simulink library "xpclib"  (Simulink 6.0)
settings: Solver=ode45  SolverMode=SingleTasking  StartTime=0.0  StopTime=10.0  RelTol=1e-3
values from neighbouring files (symbols this model uses):
  base = get_param( gcb, 'base' )    [maddiamondmm.m]    (also in maddiamondmm32frame.m; maddsmm16at.m; mdadsmm16at.m; mdiortddm64x0.m = hex2dec(addr(3:end)))
  block = find_system(bdroot,                          'FollowLinks', 'on',                          'LookUnderMasks', 'all',                          'MaskType', type )    [mdionipci6527.m]
  count = count + 1    (= 5)    [mdecodestate.m]
  port = get_param( gcb, 'port' )    [mdionipci6527.m]    (also in mdiortddm64x0.m = get_param(blocks{i}, 'port'))
undefined symbols (not defined in the file or in its folder): CIO, devid, DIO24, genixlib, get, handlers, irq, mbaseserialmask, mbwaudpmc, mdacbpcidas, mdiamondemeraldmask, mgenix, mmodemcontrol, mquamask, mrs232, msc150checks, mtargetboxleds, mtargetboxwatchdog, mxpccan, PCI, sizeof, vendid
libraries: xpclib x384, simulink x6
(part 4 of 7)

== system xpclib/RS232/Diamond/Emerald-MM8  ==
  Diamond Emerald-MM8 Serial : Subsystem  InitFcn=mdiamondemeraldmask(4,8)  TreatAsAtomicUnit=on  PropExecContextAcrossSSBoundary=on  mask(RS232 Send Receive){group=Board Setup, port=1, irqnum=5, saddr1=0x200, baud1=115200, parity1=None, ndata1=8, nstop1=1, fifomode1=16 deep, rlevel1=1, automode1=on, xmtfifosize1=1024, xmtdatatype1=8 bit uint null terminated, rcvfifosize1=1024, rcvmaxread1=1024, rcvminread1=1, rcvusedelim1=on, rcvdelim1=13, rcvdatatype1=count+16 bit uint, rcvsampletime1=-1, baud2=115200, parity2=None, ndata2=8, nstop2=1, fifomode2=16 deep, rlevel2=1, automode2=on, xmtfifosize2=1024, xmtdatatype2=8 bit uint null terminated, rcvfifosize2=1024, rcvmaxread2=1024, rcvminread2=1, rcvusedelim2=on, rcvdelim2=13, rcvdatatype2=count+16 bit uint, rcvsampletime2=-1, baud3=115200, parity3=None, ndata3=8, nstop3=1, fifomode3=16 deep, rlevel3=1, automode3=on, xmtfifosize3=1024, xmtdatatype3=8 bit uint null terminated, rcvfifosize3=1024, rcvmaxread3=1024, rcvminread3=1, rcvusedelim3=on, rcvdelim3=13, rcvdatatype3=count+16 bit uint, rcvsampletime3=-1, baud4=115200, parity4=None, ndata4=8, nstop4=1, fifomode4=16 deep, rlevel4=1, automode4=on, xmtfifosize4=1024, xmtdatatype4=8 bit uint null terminated, rcvfifosize4=1024, rcvmaxread4=1024, rcvminread4=1, rcvusedelim4=on, rcvdelim4=13, rcvdatatype4=count+16 bit uint, rcvsampletime4=-1, baud5=115200, parity5=None, ndata5=8, nstop5=1, fifomode5=16 deep, rlevel5=1, automode5=on, xmtfifosize5=1024, xmtdatatype5=8 bit uint null terminated, rcvfifosize5=1024, rcvmaxread5=1024, rcvminread5=1, rcvusedelim5=on, rcvdelim5=13, rcvdatatype5=count+16 bit uint, rcvsampletime5=-1, baud6=115200, parity6=None, ndata6=8, nstop6=1, fifomode6=16 deep, rlevel6=1, automode6=on, xmtfifosize6=1024, xmtdatatype6=8 bit uint null terminated, rcvfifosize6=1024, rcvmaxread6=1024, rcvminread6=1, rcvusedelim6=on, rcvdelim6=13, rcvdatatype6=count+16 bit uint, rcvsampletime6=-1, baud7=115200, parity7=None, ndata7=8, nstop7=1, fifomode7=16 deep, rlevel7=1, automode7=on, xmtfifosize7=1024, xmtdatatype7=8 bit uint null terminated, rcvfifosize7=1024, rcvmaxread7=1024, rcvminread7=1, rcvusedelim7=on, rcvdelim7=13, rcvdatatype7=count+16 bit uint, rcvsampletime7=-1, baud8=115200, parity8=None, ndata8=8, nstop8=1, fifomode8=16 deep, rlevel8=1, automode8=on, xmtfifosize8=1024, xmtdatatype8=8 bit uint null terminated, rcvfifosize8=1024, rcvmaxread8=1024, rcvminread8=1, rcvusedelim8=on, rcvdelim8=13, rcvdatatype8=count+16 bit uint, rcvsampletime8=-1}
      mask prompts: group "Parameter group:"; port "Port to modify:"; irqnum "IRQ number:"; saddr1 "Base address:"; baud1 "Baud rate:"; parity1 "Parity:"; ndata1 "Data bits:"; nstop1 "Stop bits:"; fifomode1 "Hardware fifo size:"; rlevel1 "Receive fifo interrupt level:"; automode1 "Auto RTS/CTS:"; xmtfifosize1 "Transmit software fifo size:"; xmtdatatype1 "Transmit fifo data type:"; rcvfifosize1 "Receive software fifo size:"; rcvmaxread1 "Receive maximum read:"; rcvminread1 "Receive minimum read:"; rcvusedelim1 "Read to delimiter:"; rcvdelim1 "Delimiter:"; rcvdatatype1 "Receive data type:"; rcvsampletime1 "Receive SampleTime:"; baud2 "Baud rate:"; parity2 "Parity:"; ndata2 "Data bits:"; nstop2 "Stop bits:"; fifomode2 "Hardware fifo size:"; rlevel2 "Receive fifo interrupt level:"; automode2 "Auto RTS/CTS:"; xmtfifosize2 "Transmit software fifo size:"; xmtdatatype2 "Transmit fifo data type:"; rcvfifosize2 "Receive software fifo size:"; rcvmaxread2 "Receive maximum read:"; rcvminread2 "Receive minimum read:"; rcvusedelim2 "Read to delimiter:"; rcvdelim2 "Delimiter:"; rcvdatatype2 "Receive data type:"; rcvsampletime2 "Receive SampleTime:"; baud3 "Baud rate:"; parity3 "Parity:"; ndata3 "Data bits:"; nstop3 "Stop bits:"; fifomode3 "Hardware fifo size:"; rlevel3 "Receive fifo interrupt level:"; automode3 "Auto RTS/CTS:"; xmtfifosize3 "Transmit software fifo size:"; xmtdatatype3 "Transmit fifo data type:"; rcvfifosize3 "Receive software fifo size:"; rcvmaxread3 "Receive maximum read:"; rcvminread3 "Receive minimum read:"; rcvusedelim3 "Read to delimiter:"; rcvdelim3 "Delimiter:"; rcvdatatype3 "Receive data type:"; rcvsampletime3 "Receive SampleTime:"; baud4 "Baud rate:"; parity4 "Parity:"; ndata4 "Data bits:"; nstop4 "Stop bits:"; fifomode4 "Hardware fifo size:"; rlevel4 "Receive fifo interrupt level:"; automode4 "Auto RTS/CTS:"; xmtfifosize4 "Transmit software fifo size:"; xmtdatatype4 "Transmit fifo data type:"; rcvfifosize4 "Receive software fifo size:"; rcvmaxread4 "Receive maximum read:"; rcvminread4 "Receive minimum read:"; rcvusedelim4 "Read to delimiter:"; rcvdelim4 "Delimiter:"; rcvdatatype4 "Receive data type:"; rcvsampletime4 "Receive SampleTime:"; baud5 "Baud rate:"; parity5 "Parity:"; ndata5 "Data bits:"; nstop5 "Stop bits:"; fifomode5 "Hardware fifo size:"; rlevel5 "Receive fifo interrupt level:"; automode5 "Auto RTS/CTS:"; xmtfifosize5 "Transmit software fifo size:"; xmtdatatype5 "Transmit fifo data type:"; rcvfifosize5 "Receive software fifo size:"; rcvmaxread5 "Receive maximum read:"; rcvminread5 "Receive minimum read:"; rcvusedelim5 "Read to delimiter:"; rcvdelim5 "Delimiter:"; rcvdatatype5 "Receive data type:"; rcvsampletime5 "Receive SampleTime:"; baud6 "Baud rate:"; parity6 "Parity:"; ndata6 "Data bits:"; nstop6 "Stop bits:"; fifomode6 "Hardware fifo size:"; rlevel6 "Receive fifo interrupt level:"; automode6 "Auto RTS/CTS:"; xmtfifosize6 "Transmit software fifo size:"; xmtdatatype6 "Transmit fifo data type:"; rcvfifosize6 "Receive software fifo size:"; rcvmaxread6 "Receive maximum read:"; rcvminread6 "Receive minimum read:"; rcvusedelim6 "Read to delimiter:"; rcvdelim6 "Delimiter:"; rcvdatatype6 "Receive data type:"; rcvsampletime6 "Receive SampleTime:"; baud7 "Baud rate:"; parity7 "Parity:"; ndata7 "Data bits:"; nstop7 "Stop bits:"; fifomode7 "Hardware fifo size:"; rlevel7 "Receive fifo interrupt level:"; automode7 "Auto RTS/CTS:"; xmtfifosize7 "Transmit software fifo size:"; xmtdatatype7 "Transmit fifo data type:"; rcvfifosize7 "Receive software fifo size:"; rcvmaxread7 "Receive maximum read:"; rcvminread7 "Receive minimum read:"; rcvusedelim7 "Read to delimiter:"; rcvdelim7 "Delimiter:"; rcvdatatype7 "Receive data type:"; rcvsampletime7 "Receive SampleTime:"; baud8 "Baud rate:"; parity8 "Parity:"; ndata8 "Data bits:"; nstop8 "Stop bits:"; fifomode8 "Hardware fifo size:"; rlevel8 "Receive fifo interrupt level:"; automode8 "Auto RTS/CTS:"; xmtfifosize8 "Transmit software fifo size:"; xmtdatatype8 "Transmit fifo data type:"; rcvfifosize8 "Receive software fifo size:"; rcvmaxread8 "Receive maximum read:"; rcvminread8 "Receive minimum read:"; rcvusedelim8 "Read to delimiter:"; rcvdelim8 "Delimiter:"; rcvdatatype8 "Receive data type:"; rcvsampletime8 "Receive SampleTime:"
      mask help:
      | Diamond Emerald MM-8
      | RS232 Send Receive Subsystem
      mask init:
      | addr = mdiamondemeraldmask( 1, 8 );
      | % addr(1) is base address, not used
      | baddr1 = addr{2};
      | baddr2 = addr{3};
      | baddr3 = addr{4};
      | baddr4 = addr{5};
      | baddr5 = addr{6};
      | baddr6 = addr{7};
      | baddr7 = addr{8};
      | baddr8 = addr{9};
      | istat = addr{10};
      | mdiamondemeraldmask( 3, 8 );
      mask Help: helpview(fullfile(docroot, 'mapfiles', 'xpc.map'), 'Baseboard_Serial_Subsystem')
      mask StyleString: popup(Board Setup|Basic Setup|Transmit Setup|Receive Setup),popup(1|2|3|4|5|6|7|8),edit,popup(0x100|0x140|0x180|0x1c0|0x200|0x240|0x280|0x2c0|0c300|0x340|0x380|0x3c0),popup(115200|57600|38400|19200|9600|4800|2400|1200|600|300|110),popup(None|Even|Odd|Mark|Space),popup(5|6|7|8),popup(1|2),popup(64 deep|16 deep|1 deep),popup(1|quarter full|half full|almost full),checkbox,edit,popup(count+32 bit int|count+32 bit uint|count+16 bit int|count+16 bit uint|8 bit int null terminated|8 bit uint null terminated),edit,edit,edit,checkbox,edit,popup(count+32 bit int|count+32 bit uint|count+16 bit int|count+16 bit uint|8 bit int null terminated|8 bit uint null terminated),edit,popup(115200|57600|38400|19200|9600|4800|2400|1200|600|300|110),popup(None|Even|Odd|Mark|Space),popup(5|6|7|8),popup(1|2),popup(64 deep|16 deep|1 deep),popup(1|quarter full|half full|almost full),checkbox,edit,popup(count+32 bit int|count+32 bit uint|count+16 bit int|count+16 bit uint|8 bit int null terminated|8 bit uint null terminated),edit,edit,edit,checkbox,edit,popup(count+32 bit int|count+32 bit uint|count+16 bit int|count+16 bit uint|8 bit int null terminated|8 bit uint null terminated),edit,popup(115200|57600|38400|19200|9600|4800|2400|1200|600|300|110),popup(None|Even|Odd|Mark|Space),popup(5|6|7|8),popup(1|2),popup(64 deep|16 deep|1 deep),popup(1|quarter full|half full|almost full),checkbox,edit,popup(count+32 bit int|count+32 bit uint|count+16 bit int|count+16 bit uint|8 bit int null terminated|8 bit uint null terminated),edit,edit,edit,checkbox,edit,popup(count+32 bit int|count+32 bit uint|count+16 bit int|count+16 bit uint|8 bit int null terminated|8 bit uint null terminated),edit,popup(115200|57600|38400|19200|9600|4800|2400|1200|600|300|110),popup(None|Even|Odd|Mark|Space),popup(5|6|7|8),popup(1|2),popup(64 deep|16 deep|1 deep),popup(1|quarter full|half full|almost full),checkbox,edit,popup(count+32 bit int|count+32 bit uint|count+16 bit int|count+16 bit uint|8 bit int null terminated|8 bit uint null terminated),edit,edit,edit,checkbox,edit,popup(count+32 bit int|count+32 bit uint|count+16 bit int|count+16 bit uint|8 bit int null terminated|8 bit uint null terminated),edit,popup(115200|57600|38400|19200|9600|4800|2400|1200|600|300|110),popup(None|Even|Odd|Mark|Space),popup(5|6|7|8),popup(1|2),popup(64 deep|16 deep|1 deep),popup(1|quarter full|half full|almost full),checkbox,edit,popup(count+32 bit int|count+32 bit uint|count+16 bit int|count+16 bit uint|8 bit int null terminated|8 bit uint null terminated),edit,edit,edit,checkbox,edit,popup(count+32 bit int|count+32 bit uint|count+16 bit int|count+16 bit uint|8 bit int null terminated|8 bit uint null terminated),edit,popup(115200|57600|38400|19200|9600|4800|2400|1200|600|300|110),popup(None|Even|Odd|Mark|Space),popup(5|6|7|8),popup(1|2),popup(64 deep|16 deep|1 deep),popup(1|quarter full|half full|almost full),checkbox,edit,popup(count+32 bit int|count+32 bit uint|count+16 bit int|count+16 bit uint|8 bit int null terminated|8 bit uint null terminated),edit,edit,edit,checkbox,edit,popup(count+32 bit int|count+32 bit uint|count+16 bit int|count+16 bit uint|8 bit int null terminated|8 bit uint null terminated),edit,popup(115200|57600|38400|19200|9600|4800|2400|1200|600|300|110),popup(None|Even|Odd|Mark|Space),popup(5|6|7|8),popup(1|2),popup(64 deep|16 deep|1 deep),popup(1|quarter full|half full|almost full),checkbox,edit,popup(count+32 bit int|count+32 bit uint|count+16 bit int|count+16 bit uint|8 bit int null terminated|8 bit uint null terminated),edit,edit,edit,checkbox,edit,popup(count+32 bit int|count+32 bit uint|count+16 bit int|count+16 bit uint|8 bit int null terminated|8 bit uint null terminated),edit,popup(115200|57600|38400|19200|9600|4800|2400|1200|600|300|110),popup(None|Even|Odd|Mark|Space),popup(5|6|7|8),popup(1|2),popup(64 deep|16 deep|1 deep),popup(1|quarter full|half full|almost full),checkbox,edit,popup(count+32 bit int|count+32 bit uint|count+16 bit int|count+16 bit uint|8 bit int null terminated|8 bit uint null terminated),edit,edit,edit,checkbox,edit,popup(count+32 bit int|count+32 bit uint|count+16 bit int|count+16 bit uint|8 bit int null terminated|8 bit uint null terminated),edit
      mask CallbackString:
      | mdiamondemeraldmask( 2, 8 );
      | |mdiamondemeraldmask( 2, 8 );||||||||||||||||||||||||||||||||||||||||||||||||||||||||||||||||||||||||||||||||||||||||||||||||||||||||||||||||||||||||||||||||||
      mask Display:
      | disp('Diamond\n\nEmerald\n\nRS232\nSend Receive');
      | port_label('input',1,'XMT1');
      | port_label('input',2,'XMT2');
      | port_label('input',3,'XMT3');
      | port_label('input',4,'XMT4');
      | port_label('input',5,'XMT5');
      | port_label('input',6,'XMT6');
      | port_label('input',7,'XMT7');
      | port_label('input',8,'XMT8');
      | port_label('output',1,'RCV1');
      | port_label('output',2,'RCV2');
      | port_label('output',3,'RCV3');
      | port_label('output',4,'RCV4');
      | port_label('output',5,'RCV5');
      | port_label('output',6,'RCV6');
      | port_label('output',7,'RCV7');
      | port_label('output',8,'RCV8');
  "Diamond Emerald-MM8 " : Subsystem  PropExecContextAcrossSSBoundary=on
  "Modem Control " : S-Function  InitFcn=mmodemcontrol(5);  FunctionName=modemcontrolemeraldmm  Parameters=addr, boardtype, rts, dtr, count  mask(Modem Control){port=1, rts=on, dtr=on, firstaddr=0x200}
      mask prompts: firstaddr "Configuration port address:"
      mask help:
      | Diamond Emerald-MM-8
      | Modem Control
      mask init:
      | count = 0;
      | boardtype = 6;
      | [maskdisplay, count, addr] = mmodemcontrol( 2, rts, dtr, boardtype, port, firstaddr );
      | addr = hex2dec( addr(3:end) );
      | set_param( gcb, 'MaskDisplay', maskdisplay );
      mask Help: helpview(fullfile(docroot, 'mapfiles', 'xpc.map'), 'Emerald_MODEM_Control')
      mask StyleString: popup(1|2|3|4|5|6|7|8),checkbox,checkbox,popup(0x100|0x140|0x180|0x1c0|0x200|0x240|0x280|0x2c0|0x300|0x340|0x380|0x3c0)
      mask Display: disp('Diamond\nEmerald-MM-8\nModem Control');port_label('input',1,'RTS');port_label('input',2,'DTR');
  "Modem Status " : S-Function  FunctionName=modemstatusemeraldmm  Parameters=addr, boardtype, cts, dsr, ring, dcd, count, sampletime  mask(Modem Status){port=1, cts=on, dsr=on, ring=on, dcd=on, sampletime=-1, firstaddr=0x200}
      mask prompts: ring "RI:"; firstaddr "Configuration port address:"
      mask help:
      | Diamond Emerald-MM-8
      | Modem Status
      mask init:
      | count = 0;
      | boardtype = 6;
      | [maskdisplay, count, addr] = mmodemstatus( 2, cts, dsr, ring, dcd, boardtype, port, firstaddr );
      | addr = hex2dec( addr(3:end) );
      | set_param( gcb, 'MaskDisplay', maskdisplay );
      mask Help: helpview(fullfile(docroot, 'mapfiles', 'xpc.map'), 'Emerald_MODEM_Status')
      mask StyleString: popup(1|2|3|4|5|6|7|8),checkbox,checkbox,checkbox,checkbox,edit,popup(0x100|0x140|0x180|0x1c0|0x200|0x240|0x280|0x2c0|0x300|0x340|0x380|0x3c0)
      mask Display: disp('Diamond\nEmerald-MM-8\nModem Status');port_label('output',1,'CTS');port_label('output',2,'DSR');port_label('output',3,'RI');port_label('output',4,'DCD');

== system xpclib/RS232/Mainboard/Baseboard Serial ==
  In1 : Inport  LatchInput=off
  In2 : Inport  Port=2  LatchInput=off
  Async Rate Transition{,1..3} (4 alike) : xpclib/Asynchronous Event/Async Rate Transition  sample_time=-1
  Enable TX 1 : xpclib/RS232/Mainboard/Baseboard Serial Internal  blocks/Enable TX   addr=baddr1
  Enable TX 2 : xpclib/RS232/Mainboard/Baseboard Serial Internal  blocks/Enable TX   addr=baddr2
  FIFO read 1 : xpclib/RS232/FIFO read   maxsize=1024  minsize=1  usedelimiter=on  delimiter=13  outputtype=count+16 bit uint  enable=off  enableout=off  sampletime=-1
  FIFO read 2 : xpclib/RS232/FIFO read   maxsize=1024  minsize=1  usedelimiter=on  delimiter=13  outputtype=count+16 bit uint  enable=off  enableout=off  sampletime=-1
  FIFO write 1 : xpclib/RS232/FIFO write   size=1024  inputtype=8 bit uint null terminated  present=on  sampletime=-1  id=XMT channel 1, IRQ 4
  FIFO write 2 : xpclib/RS232/FIFO write   size=1024  inputtype=8 bit uint null terminated  present=on  sampletime=-1  id=XMT channel 2, IRQ 4
  IRQ Source : xpclib/Asynchronous Event/IRQ Source  irqNo=4  preempt=off  b_type=None/Other  slot=-1
  RS232 ISR : Subsystem  TreatAsAtomicUnit=on  PropExecContextAcrossSSBoundary=on  mask(RS232 ISR){addr1=baddr1, addr2=baddr2}
      mask prompts: addr1 "First channel address:"; addr2 "Second channel address:"
      mask help:
      | Baseboard Serial
      | Interrupt Service Routine
      mask init:
      | baddr1 = addr1;
      | baddr2 = addr2;
      mask Display:
      | disp('Baseboard\nSerial\nISR');
      | port_label('input', 1, 'XMT1');
      | port_label('input', 2, 'XMT3');
      | port_label('output', 1, 'RCV1');
      | port_label('output', 2, 'RCV3');
  Setup1 : xpclib/RS232/Mainboard/Baseboard Serial Internal  blocks/Setup  baud=115200  width=8  nstop=1  parity=None  fmode=16 deep  rlevel=half full  ctsmode=on  addr=baddr1
  Setup2 : xpclib/RS232/Mainboard/Baseboard Serial Internal  blocks/Setup  baud=115200  width=8  nstop=1  parity=None  fmode=16 deep  rlevel=half full  ctsmode=off  addr=baddr2
  Out1 : Outport
  Out2 : Outport  Port=2
  wires:
  Async Rate Transition3/1 -> RS232 ISR/2(Xmt 2)
  FIFO write 2/2 -> Enable TX 2/1
  FIFO read 2/1 -> Out2/1
  Async Rate Transition1/1 -> FIFO read 2/1
  FIFO read 1/1 -> Out1/1
  Async Rate Transition/1 -> FIFO read 1/1
  In2/1 -> FIFO write 2/1
  FIFO write 2/1 -> Async Rate Transition3/1
  In1/1 -> FIFO write 1/1
  FIFO write 1/1 -> Async Rate Transition2/1
  RS232 ISR/2(Recv 2) -> Async Rate Transition1/1
  RS232 ISR/1(Recv 1) -> Async Rate Transition/1
  Async Rate Transition2/1 -> RS232 ISR/1(Xmt 1)
  IRQ Source/1 -> RS232 ISR/Trigger
  FIFO write 1/2 -> Enable TX 1/1

== system xpclib/RS232/Mainboard/Baseboard Serial Internal  blocks ==
  "Enable TX " : S-Function  FunctionName=sertxenablebase  Parameters=addr  mask(Enable TX Int){addr=0}
      mask prompts: addr "Base address:"
      mask help:
      | Baseboard Serial
      | Enable TX Interrupt
      mask init:
      | addr = hex2dec( addr(3:end) );
      mask Help: helpview(fullfile(docroot, 'mapfiles', 'xpc.map'), 'Baseboard_Enable_Int')
      mask Display:
      | disp('Baseboard\nSerial\nEnable TX Int');
      | port_label('input', 1, 'E');
  Filter Int Reason : S-Function  FunctionName=filterserint  Parameters=port, value  mask(Interrupt Source Filter){port=1, value=Receive data}
      mask prompts: value "Filter value:"
      mask help:
      | Baseboard
      | Interrupt Source Filter
      mask Help: helpview(fullfile(docroot, 'mapfiles', 'xpc.map'), 'Baseboard_Filter_Ints')
      mask StyleString: popup(1|2),popup(Receive data|Transmitter empty|Modem status change)
      mask Display:
      | disp('Baseboard\nSerial\nFilter Int Reason');
      | port_label('input', 1, 'S' );
      | port_label('output', 1, 'E' );
  Read HW FIFO : S-Function  FunctionName=serreadbase  Parameters=addr, flush  mask(Read Data Port){flush=on, addr=0}
      mask prompts: flush "Flush HW FIFO on startup"; addr "Base address:"
      mask help:
      | Baseboard
      | Read Data Port
      mask init:
      | addr = hex2dec( addr(3:end) );
      mask Help: helpview(fullfile(docroot, 'mapfiles', 'xpc.map'), 'Baseboard_Read_HW')
      mask Display:
      | disp('Baseboard\nSerial\nRead HW FIFO');
      | port_label('input', 1, 'E');
      | port_label('output', 1, 'D');
  Read Int Status : S-Function  FunctionName=iquerybase  Parameters=addr1, addr2  mask(Interrupt Query){addr1=0, addr2=0}
      mask prompts: addr1 "Base address 1"; addr2 "Base address 2"
      mask help:
      | Baseboard Serial
      | Interrupt Query
      mask init:
      | addr1 = hex2dec( addr1(3:end) );
      | addr2 = hex2dec( addr2(3:end) );
      mask Help: helpview(fullfile(docroot, 'mapfiles', 'xpc.map'), 'Baseboard_Interrupt_Query')
      mask Display:
      | disp('Baseboard\nSerial\nRead Int Status');
      | port_label('output', 1, 'S' );
  Setup : S-Function  FunctionName=sersetupbase  Parameters=addr, baud, width, nstop, parity, fmode, ctsmode, rlevel  mask(setup){baud=115200, width=8, nstop=1, parity=None, fmode=16 deep, rlevel=half full, ctsmode=off, addr=0}
      mask prompts: baud "Baud rate:"; width "Number of data bits:"; nstop "Number of stop bits:"; fmode "Fifo mode:"; rlevel "Receive trigger level:"; ctsmode "Enable auto RTS/CTS"; addr "Base Address:"
      mask help:
      | Baseboard
      | Serial
      | Setup
      mask init:
      | addr = hex2dec( addr(3:end) );
      mask Help: helpview(fullfile(docroot, 'mapfiles', 'xpc.map'), 'Baseboard_Setup')
      mask StyleString: popup(115200|57600|38400|19200|9600|4800|2400|1200|600|300|110),popup(5|6|7|8),popup(1|2),popup(None|Even|Odd|Mark|Space),popup(64 deep|16 deep|1 deep),popup(1|quarter full|half full|almost full),checkbox,edit
      mask Display: disp('Baseboard\nSerial\nSetup');
  Write HW FIFO : S-Function  FunctionName=serwritebase  Parameters=addr  mask(Write Data Port){addr=0}
      mask prompts: addr "Base address:"
      mask help:
      | Baseboard
      | Write Data Port
      mask init:
      | addr = hex2dec( addr(3:end) );
      mask Help: helpview(fullfile(docroot, 'mapfiles', 'xpc.map'), 'Baseboard_Write_HW')
      mask Display:
      | disp('Baseboard\nSerial\nWrite HW FIFO');
      | port_label('input', 1, 'D');
      | port_label('input', 2, 'E');

== system xpclib/RS232/Quatech/ESC-100 ==
  ESC-100 : Subsystem  InitFcn=mquamask(3)  TreatAsAtomicUnit=on  PropExecContextAcrossSSBoundary=on  mask(ESC-100 RS232 Send Receive){group=Board Setup, port=1, irqnum=7, slot=-1, baud1=19200, parity1=None, ndata1=8, nstop1=1, fifomode1=64 deep, rlevel1=half full, automode1=on, xmtfifosize1=1024, xmtdatatype1=8 bit uint null terminated, rcvfifosize1=1024, rcvmaxread1=1024, rcvminread1=1, rcvusedelim1=on, rcvdelim1=13, rcvdatatype1=count+16 bit uint, rcvsampletime1=-1, baud2=19200, parity2=None, ndata2=8, nstop2=1, fifomode2=64 deep, rlevel2=half full, automode2=on, xmtfifosize2=1024, xmtdatatype2=8 bit uint null terminated, rcvfifosize2=1024, rcvmaxread2=1024, rcvminread2=1, rcvusedelim2=on, rcvdelim2=13, rcvdatatype2=count+16 bit uint, rcvsampletime2=-1, baud3=19200, parity3=None, ndata3=8, nstop3=1, fifomode3=64 deep, rlevel3=half full, automode3=on, xmtfifosize3=1024, xmtdatatype3=8 bit uint null terminated, rcvfifosize3=1024, rcvmaxread3=1024, rcvminread3=1, rcvusedelim3=on, rcvdelim3=13, rcvdatatype3=count+16 bit uint, rcvsampletime3=-1, buad4=19200, parity4=None, ndata4=8, nstop4=1, fifomode4=64 deep, rlevel4=half full, automode4=on, xmtfifosize4=1024, xmtdatatype4=8 bit uint null terminated, rcvfifosize4=1024, rcvmaxread4=1024, rcvminread4=1, rcvusedelim4=on, rcvdelim4=13, rcvdatatype4=count+16 bit uint, rcvsampletime4=-1, baud5=19200, parity5=None, ndata5=8, nstop5=1, fifomode5=64 deep, rlevel5=half full, automode5=on, xmtfifosize5=1024, xmtdatatype5=8 bit uint null terminated, rcvfifosize5=1024, rcvmaxread5=1024, rcvminread5=1, rcvusedelim5=on, rcvdelim5=13, rcvdatatype5=count+16 bit uint, rcvsampletime5=-1, baud6=19200, parity6=None, ndata6=8, nstop6=1, fifomode6=64 deep, rlevel6=half full, automode6=on, xmtfifosize6=1024, xmtdatatype6=8 bit uint null terminated, rcvfifosize6=1024, rcvmaxread6=1024, rcvminread6=1, rcvusedelim6=on, rcvdelim6=13, rcvdatatype6=count+16 bit uint, rcvsampletime6=-1, baud7=19200, parity7=None, ndata7=8, nstop7=1, fifomode7=64 deep, rlevel7=half full, automode7=on, xmtfifosize7=1024, xmtdatatype7=8 bit uint null terminated, rcvfifosize7=1024, rcvmaxread7=1024, rcvminread7=1, rcvusedelim7=on, rcvdelim7=13, rcvdatatype7=count+16 bit uint, rcvsampletime7=-1, baud8=19200, parity8=None, ndata8=8, nstop8=1, fifomode8=64 deep, rlevel8=half full, automode8=on, xmtfifosize8=1024, xmtdatatype8=8 bit uint null terminated, rcvfifosize8=1024, rcvmaxread8=1024, rcvminread8=1, rcvusedelim8=on, rcvdelim8=13, rcvdatatype8=count+16 bit uint, rcvsampletime8=-1}
      mask prompts: group "Parameter group:"; port "Port to modify:"; irqnum "IRQ number:"; baud1 "Baud rate:"; parity1 "Parity:"; ndata1 "Data bits:"; nstop1 "Stop bits:"; fifomode1 "Hardware fifo size:"; rlevel1 "Receive fifo interrupt level:"; automode1 "Auto RTS/CTS:"; xmtfifosize1 "Transmit software fifo size:"; xmtdatatype1 "Transmit fifo data type:"; rcvfifosize1 "Receive software fifo size:"; rcvmaxread1 "Receive maximum read:"; rcvminread1 "Receive minimum read:"; rcvusedelim1 "Read to delimiter:"; rcvdelim1 "Delimiter:"; rcvdatatype1 "Receive data type:"; rcvsampletime1 "Receive SampleTime:"; baud2 "Baud rate:"; parity2 "Parity:"; ndata2 "Data bits:"; nstop2 "Stop bits:"; fifomode2 "Hardware fifo size:"; rlevel2 "Receive fifo interrupt level:"; automode2 "Auto RTS/CTS:"; xmtfifosize2 "Transmit software fifo size:"; xmtdatatype2 "Transmit fifo data type:"; rcvfifosize2 "Receive software fifo size:"; rcvmaxread2 "Receive maximum read:"; rcvminread2 "Receive minimum read:"; rcvusedelim2 "Read to delimiter:"; rcvdelim2 "Delimiter:"; rcvdatatype2 "Receive data type:"; rcvsampletime2 "Receive SampleTime:"; baud3 "Baud rate:"; parity3 "Parity:"; ndata3 "Data bits:"; nstop3 "Stop bits:"; fifomode3 "Hardware fifo size:"; rlevel3 "Receive fifo interrupt level:"; automode3 "Auto RTS/CTS:"; xmtfifosize3 "Transmit software fifo size:"; xmtdatatype3 "Transmit fifo data type:"; rcvfifosize3 "Receive software fifo size:"; rcvmaxread3 "Receive maximum read:"; rcvminread3 "Receive minimum read:"; rcvusedelim3 "Read to delimiter:"; rcvdelim3 "Delimiter:"; rcvdatatype3 "Receive data type:"; rcvsampletime3 "Receive SampleTime:"; buad4 "Baud rate:"; parity4 "Parity:"; ndata4 "Data bits:"; nstop4 "Stop bits:"; fifomode4 "Hardware fifo size:"; rlevel4 "Receive fifo interrupt level:"; automode4 "Auto RTS/CTS:"; xmtfifosize4 "Transmit software fifo size:"; xmtdatatype4 "Transmit fifo data type:"; rcvfifosize4 "Receive software fifo size:"; rcvmaxread4 "Receive maximum read:"; rcvminread4 "Receive minimum read:"; rcvusedelim4 "Read to delimiter:"; rcvdelim4 "Delimiter:"; rcvdatatype4 "Receive data type:"; rcvsampletime4 "Receive SampleTime:"; baud5 "Baud rate:"; parity5 "Parity:"; ndata5 "Data bits:"; nstop5 "Stop bits:"; fifomode5 "Hardware fifo size:"; rlevel5 "Receive fifo interrupt level:"; automode5 "Auto RTS/CTS:"; xmtfifosize5 "Transmit software fifo size:"; xmtdatatype5 "Transmit fifo data type:"; rcvfifosize5 "Receive software fifo size:"; rcvmaxread5 "Receive maximum read:"; rcvminread5 "Receive minimum read:"; rcvusedelim5 "Read to delimiter:"; rcvdelim5 "Delimiter:"; rcvdatatype5 "Receive data type:"; rcvsampletime5 "Receive SampleTime:"; baud6 "Baud rate:"; parity6 "Parity:"; ndata6 "Data bits:"; nstop6 "Stop bits:"; fifomode6 "Hardware fifo size:"; rlevel6 "Receive fifo interrupt level:"; automode6 "Auto RTS/CTS:"; xmtfifosize6 "Transmit software fifo size:"; xmtdatatype6 "Transmit fifo data type:"; rcvfifosize6 "Receive software fifo size:"; rcvmaxread6 "Receive maximum read:"; rcvminread6 "Receive minimum read:"; rcvusedelim6 "Read to delimiter:"; rcvdelim6 "Delimiter:"; rcvdatatype6 "Receive data type:"; rcvsampletime6 "Receive SampleTime:"; baud7 "Baud rate:"; parity7 "Parity:"; ndata7 "Data bits:"; nstop7 "Stop bits:"; fifomode7 "Hardware fifo size:"; rlevel7 "Receive fifo interrupt level:"; automode7 "Auto RTS/CTS:"; xmtfifosize7 "Transmit software fifo size:"; xmtdatatype7 "Transmit fifo data type:"; rcvfifosize7 "Receive software fifo size:"; rcvmaxread7 "Receive maximum read:"; rcvminread7 "Receive minimum read:"; rcvusedelim7 "Read to delimiter:"; rcvdelim7 "Delimiter:"; rcvdatatype7 "Receive data type:"; rcvsampletime7 "Receive SampleTime:"; baud8 "Baud rate:"; parity8 "Parity:"; ndata8 "Data bits:"; nstop8 "Stop bits:"; fifomode8 "Hardware fifo size:"; rlevel8 "Receive fifo interrupt level:"; automode8 "Auto RTS/CTS:"; xmtfifosize8 "Transmit software fifo size:"; xmtdatatype8 "Transmit fifo data type:"; rcvfifosize8 "Receive software fifo size:"; rcvmaxread8 "Receive maximum read:"; rcvminread8 "Receive minimum read:"; rcvusedelim8 "Read to delimiter:"; rcvdelim8 "Delimiter:"; rcvdatatype8 "Receive data type:"; rcvsampletime8 "Receive SampleTime:"
      mask help:
      | ESC-100
      | Quatech
      | RS232 Send Receive Subsystem
      mask init:
      | brdslot = slot;
      | mquamask( 1, 8 );
      mask Help: helpview(fullfile(docroot, 'mapfiles', 'xpc.map'), 'Quatech_Subsystem')
      mask StyleString: popup(Board Setup|Basic Setup|Transmit Setup|Receive Setup),popup(1|2|3|4|5|6|7|8),edit,edit,popup(921600|460800|230400|115200|57600|38400|19200|9600|4800|2400|1200|600|300|110),popup(None|Even|Odd|Mark|Space),popup(5|6|7|8),popup(1|2),popup(64 deep|16 deep|1 deep),popup(1|quarter full|half full|almost full),checkbox,edit,popup(count+32 bit int|count+32 bit uint|count+16 bit int|count+16 bit uint|8 bit int null terminated|8 bit uint null terminated),edit,edit,edit,checkbox,edit,popup(count+32 bit int|count+32 bit uint|count+16 bit int|count+16 bit uint|8 bit int null terminated|8 bit uint null terminated),edit,popup(921600|460800|230400|115200|57600|38400|19200|9600|4800|2400|1200|600|300|110),popup(None|Even|Odd|Mark|Space),popup(5|6|7|8),popup(1|2),popup(64 deep|16 deep|1 deep),popup(1|quarter full|half full|almost full),checkbox,edit,popup(count+32 bit int|count+32 bit uint|count+16 bit int|count+16 bit uint|8 bit int null terminated|8 bit uint null terminated),edit,edit,edit,checkbox,edit,popup(count+32 bit int|count+32 bit uint|count+16 bit int|count+16 bit uint|8 bit int null terminated|8 bit uint null terminated),edit,popup(921600|460800|230400|115200|57600|38400|19200|9600|4800|2400|1200|600|300|110),popup(None|Even|Odd|Mark|Space),popup(5|6|7|8),popup(1|2),popup(64 deep|16 deep|1 deep),popup(1|quarter full|half full|almost full),checkbox,edit,popup(count+32 bit int|count+32 bit uint|count+16 bit int|count+16 bit uint|8 bit int null terminated|8 bit uint null terminated),edit,edit,edit,checkbox,edit,popup(count+32 bit int|count+32 bit uint|count+16 bit int|count+16 bit uint|8 bit int null terminated|8 bit uint null terminated),edit,popup(921600|460800|230400|115200|57600|38400|19200|9600|4800|2400|1200|600|300|110),popup(None|Even|Odd|Mark|Space),popup(5|6|7|8),popup(1|2),popup(64 deep|16 deep|1 deep),popup(1|quarter full|half full|almost full),checkbox,edit,popup(count+32 bit int|count+32 bit uint|count+16 bit int|count+16 bit uint|8 bit int null terminated|8 bit uint null terminated),edit,edit,edit,checkbox,edit,popup(count+32 bit int|count+32 bit uint|count+16 bit int|count+16 bit uint|8 bit int null terminated|8 bit uint null terminated),edit,popup(921600|460800|230400|115200|57600|38400|19200|9600|4800|2400|1200|600|300|110),popup(None|Even|Odd|Mark|Space),popup(5|6|7|8),popup(1|2),popup(64 deep|16 deep|1 deep),popup(1|quarter full|half full|almost full),checkbox,edit,popup(count+32 bit int|count+32 bit uint|count+16 bit int|count+16 bit uint|8 bit int null terminated|8 bit uint null terminated),edit,edit,edit,checkbox,edit,popup(count+32 bit int|count+32 bit uint|count+16 bit int|count+16 bit uint|8 bit int null terminated|8 bit uint null terminated),edit,popup(921600|460800|230400|115200|57600|38400|19200|9600|4800|2400|1200|600|300|110),popup(None|Even|Odd|Mark|Space),popup(5|6|7|8),popup(1|2),popup(64 deep|16 deep|1 deep),popup(1|quarter full|half full|almost full),checkbox,edit,popup(count+32 bit int|count+32 bit uint|count+16 bit int|count+16 bit uint|8 bit int null terminated|8 bit uint null terminated),edit,edit,edit,checkbox,edit,popup(count+32 bit int|count+32 bit uint|count+16 bit int|count+16 bit uint|8 bit int null terminated|8 bit uint null terminated),edit,popup(921600|460800|230400|115200|57600|38400|19200|9600|4800|2400|1200|600|300|110),popup(None|Even|Odd|Mark|Space),popup(5|6|7|8),popup(1|2),popup(64 deep|16 deep|1 deep),popup(1|quarter full|half full|almost full),checkbox,edit,popup(count+32 bit int|count+32 bit uint|count+16 bit int|count+16 bit uint|8 bit int null terminated|8 bit uint null terminated),edit,edit,edit,checkbox,edit,popup(count+32 bit int|count+32 bit uint|count+16 bit int|count+16 bit uint|8 bit int null terminated|8 bit uint null terminated),edit,popup(921600|460800|230400|115200|57600|38400|19200|9600|4800|2400|1200|600|300|110),popup(None|Even|Odd|Mark|Space),popup(5|6|7|8),popup(1|2),popup(64 deep|16 deep|1 deep),popup(1|quarter full|half full|almost full),checkbox,edit,popup(count+32 bit int|count+32 bit uint|count+16 bit int|count+16 bit uint|8 bit int null terminated|8 bit uint null terminated),edit,edit,edit,checkbox,edit,popup(count+32 bit int|count+32 bit uint|count+16 bit int|count+16 bit uint|8 bit int null terminated|8 bit uint null terminated),edit
      mask CallbackString:
      | mquamask( 2, 8 );
      | |mquamask( 2, 8 );||||||||||||||||||||||||||||||||||||||||||||||||||||||||||||||||||||||||||||||||||||||||||||||||||||||||||||||||||||||||||||||||||
      mask Display:
      | disp('ESC-100\n\nRS232\n\nSend Receive');
      | port_label( 'input', 1, 'XMT1' );
      | port_label( 'input', 2, 'XMT2' );
      | port_label( 'input', 3, 'XMT3' );
      | port_label( 'input', 4, 'XMT4' );
      | port_label( 'input', 5, 'XMT5' );
      | port_label( 'input', 6, 'XMT6' );
      | port_label( 'input', 7, 'XMT7' );
      | port_label( 'input', 8, 'XMT8' );
      | port_label( 'output', 1, 'RCV1' );
      | port_label( 'output', 2, 'RCV2' );
      | port_label( 'output', 3, 'RCV3' );
      | port_label( 'output', 4, 'RCV4' );
      | port_label( 'output', 5, 'RCV5' );
      | port_label( 'output', 6, 'RCV6' );
      | port_label( 'output', 7, 'RCV7' );
      | port_label( 'output', 8, 'RCV8' );
  ESC-100 Internal blocks : Subsystem  PropExecContextAcrossSSBoundary=on
  Modem Control : S-Function  InitFcn=mmodemcontrol(3)  FunctionName=modemcontrolqua  Parameters=slot, port, boardtype, rts, dtr, count  mask(ESC-100 Modem Control){port=1, rts=on, dtr=on, slot=-1}
      mask prompts: slot "PCI slot: (-1 for autosearch)"
      mask help:
      | ESC-100
      | Quatech
      | Modem Control
      mask init:
      | count = 0;
      | boardtype = 2;
      | [maskdisplay, count] = mmodemcontrol( 2, rts, dtr, boardtype, 0, 0 );
      | set_param( gcb, 'MaskDisplay', maskdisplay );
      mask Help: helpview(fullfile(docroot, 'mapfiles', 'xpc.map'), 'Quatech_MODEM_Control')
      mask StyleString: popup(1|2|3|4|5|6|7|8),checkbox,checkbox,edit
      mask Display: disp('ESC-100\nQuatech\nModem Control');port_label('input',1,'RTS');port_label('input',2,'DTR');
  Modem Status : S-Function  FunctionName=modemstatusqua  Parameters=slot, port, boardtype, cts, dsr, ring, dcd, count, sampletime  mask(Modem Status){port=1, cts=on, dsr=on, ring=on, dcd=on, sampletime=-1, slot=-1}
      mask prompts: ring "RI:"; slot "PCI slot: (-1 for autosearch)"
      mask help:
      | ESC-100
      | Quatech
      | Modem Status
      mask init:
      | count = 0;
      | boardtype = 2;
      | [maskdisplay, count] = mmodemstatus( 2, cts, dsr, ring, dcd, boardtype );
      | set_param( gcb, 'MaskDisplay', maskdisplay );
      mask Help: helpview(fullfile(docroot, 'mapfiles', 'xpc.map'), 'Quatech_MODEM_Status')
      mask StyleString: popup(1|2|3|4|5|6|7|8),checkbox,checkbox,checkbox,checkbox,edit,edit
      mask Display: disp('ESC-100\nQuatech\nModem Status');port_label('output',1,'CTS');port_label('output',2,'DSR');port_label('output',3,'RI');port_label('output',4,'DCD');

== system xpclib/RS232/Quatech/QSC-100 ==
  Modem Control : S-Function  InitFcn=mmodemcontrol(3)  FunctionName=modemcontrolqua  Parameters=slot, port, boardtype, rts, dtr, count  mask(QSC-100 Modem Control){port=1, rts=on, dtr=on, slot=-1}
      mask prompts: slot "PCI slot: (-1 for autosearch)"
      mask help:
      | QSC-100
      | Quatech
      | Modem Control
      mask init:
      | count = 0;
      | boardtype = 1;
      | [maskdisplay, count] = mmodemcontrol( 2, rts, dtr, boardtype, 0, 0 );
      | set_param( gcb, 'MaskDisplay', maskdisplay );
      mask Help: helpview(fullfile(docroot, 'mapfiles', 'xpc.map'), 'Quatech_MODEM_Control')
      mask StyleString: popup(1|2|3|4),checkbox,checkbox,edit
      mask Display: disp('QSC-100\nQuatech\nModem Control');port_label('input',1,'RTS');port_label('input',2,'DTR');
  Modem Status : S-Function  FunctionName=modemstatusqua  Parameters=slot, port, boardtype, cts, dsr, ring, dcd, count, sampletime  mask(Modem Status){port=1, cts=on, dsr=on, ring=on, dcd=on, sampletime=-1, slot=-1}
      mask prompts: ring "RI:"; slot "PCI slot: (-1 for autosearch)"
      mask help:
      | QSC-100
      | Quatech
      | Modem Status
      mask init:
      | count = 0;
      | boardtype = 1;
      | [maskdisplay, count] = mmodemstatus( 2, cts, dsr, ring, dcd, boardtype );
      | set_param( gcb, 'MaskDisplay', maskdisplay );
      mask Help: helpview(fullfile(docroot, 'mapfiles', 'xpc.map'), 'Quatech_MODEM_Status')
      mask StyleString: popup(1|2|3|4),checkbox,checkbox,checkbox,checkbox,edit,edit
      mask Display: disp('QSC-100\nQuatech\nModem Status');port_label('output',1,'CTS');port_label('output',2,'DSR');port_label('output',3,'RI');port_label('output',4,'DCD');
  QSC-100 : Subsystem  InitFcn=mquamask(3)  TreatAsAtomicUnit=on  PropExecContextAcrossSSBoundary=on  mask(QSC-100 RS232 Send Receive){group=Transmit Setup, port=1, irqnum=7, slot=-1, baud1=115200, parity1=None, ndata1=8, nstop1=1, fifomode1=64 deep, rlevel1=half full, automode1=on, xmtfifosize1=1024, xmtdatatype1=8 bit uint null terminated, rcvfifosize1=1024, rcvmaxread1=1024, rcvminread1=1, rcvusedelim1=on, rcvdelim1=13, rcvdatatype1=count+16 bit uint, rcvsampletime1=-1, baud2=115200, parity2=None, ndata2=8, nstop2=1, fifomode2=64 deep, rlevel2=half full, automode2=on, xmtfifosize2=1024, xmtdatatype2=8 bit uint null terminated, rcvfifosize2=1024, rcvmaxread2=1024, rcvminread2=1, rcvusedelim2=on, rcvdelim2=13, rcvdatatype2=count+16 bit uint, rcvsampletime2=-1, baud3=115200, parity3=None, ndata3=8, nstop3=1, fifomode3=64 deep, rlevel3=half full, automode3=on, xmtfifosize3=1024, xmtdatatype3=8 bit uint null terminated, rcvfifosize3=1024, rcvmaxread3=1024, rcvminread3=1, rcvusedelim3=on, rcvdelim3=13, rcvdatatype3=count+16 bit uint, rcvsampletime3=-1, buad4=115200, parity4=None, ndata4=8, nstop4=1, fifomode4=64 deep, rlevel4=half full, automode4=on, xmtfifosize4=1024, xmtdatatype4=8 bit uint null terminated, rcvfifosize4=1024, rcvmaxread4=1024, rcvminread4=1, rcvusedelim4=on, rcvdelim4=13, rcvdatatype4=count+16 bit uint, rcvsampletime4=-1}
      mask prompts: group "Parameter group:"; port "Port to modify:"; irqnum "IRQ number:"; baud1 "Baud rate:"; parity1 "Parity:"; ndata1 "Data bits:"; nstop1 "Stop bits:"; fifomode1 "Hardware fifo size:"; rlevel1 "Receive fifo interrupt level:"; automode1 "Auto RTS/CTS:"; xmtfifosize1 "Transmit software fifo size:"; xmtdatatype1 "Transmit fifo data type:"; rcvfifosize1 "Receive software fifo size:"; rcvmaxread1 "Receive maximum read:"; rcvminread1 "Receive minimum read:"; rcvusedelim1 "Read to delimiter:"; rcvdelim1 "Delimiter:"; rcvdatatype1 "Receive data type:"; rcvsampletime1 "Receive SampleTime:"; baud2 "Baud rate:"; parity2 "Parity:"; ndata2 "Data bits:"; nstop2 "Stop bits:"; fifomode2 "Hardware fifo size:"; rlevel2 "Receive fifo interrupt level:"; automode2 "Auto RTS/CTS:"; xmtfifosize2 "Transmit software fifo size:"; xmtdatatype2 "Transmit fifo data type:"; rcvfifosize2 "Receive software fifo size:"; rcvmaxread2 "Receive maximum read:"; rcvminread2 "Receive minimum read:"; rcvusedelim2 "Read to delimiter:"; rcvdelim2 "Delimiter:"; rcvdatatype2 "Receive data type:"; rcvsampletime2 "Receive SampleTime:"; baud3 "Baud rate:"; parity3 "Parity:"; ndata3 "Data bits:"; nstop3 "Stop bits:"; fifomode3 "Hardware fifo size:"; rlevel3 "Receive fifo interrupt level:"; automode3 "Auto RTS/CTS:"; xmtfifosize3 "Transmit software fifo size:"; xmtdatatype3 "Transmit fifo data type:"; rcvfifosize3 "Receive software fifo size:"; rcvmaxread3 "Receive maximum read:"; rcvminread3 "Receive minimum read:"; rcvusedelim3 "Read to delimiter:"; rcvdelim3 "Delimiter:"; rcvdatatype3 "Receive data type:"; rcvsampletime3 "Receive SampleTime:"; buad4 "Baud rate:"; parity4 "Parity:"; ndata4 "Data bits:"; nstop4 "Stop bits:"; fifomode4 "Hardware fifo size:"; rlevel4 "Receive fifo interrupt level:"; automode4 "Auto RTS/CTS:"; xmtfifosize4 "Transmit software fifo size:"; xmtdatatype4 "Transmit fifo data type:"; rcvfifosize4 "Receive software fifo size:"; rcvmaxread4 "Receive maximum read:"; rcvminread4 "Receive minimum read:"; rcvusedelim4 "Read to delimiter:"; rcvdelim4 "Delimiter:"; rcvdatatype4 "Receive data type:"; rcvsampletime4 "Receive SampleTime:"
      mask help:
      | QSC-100
      | Quatech
      | RS232 Send Receive Subsystem
      mask init:
      | brdslot = slot;
      | mquamask( 1, 4 );
      mask Help: helpview(fullfile(docroot, 'mapfiles', 'xpc.map'), 'Quatech_Subsystem')
      mask StyleString: popup(Board Setup|Basic Setup|Transmit Setup|Receive Setup),popup(1|2|3|4),edit,edit,popup(921600|460800|230400|115200|57600|38400|19200|9600|4800|2400|1200|600|300|110),popup(None|Even|Odd|Mark|Space),popup(5|6|7|8),popup(1|2),popup(64 deep|16 deep|1 deep),popup(1|quarter full|half full|almost full),checkbox,edit,popup(count+32 bit int|count+32 bit uint|count+16 bit int|count+16 bit uint|8 bit int null terminated|8 bit uint null terminated),edit,edit,edit,checkbox,edit,popup(count+32 bit int|count+32 bit uint|count+16 bit int|count+16 bit uint|8 bit int null terminated|8 bit uint null terminated),edit,popup(921600|460800|230400|115200|57600|38400|19200|9600|4800|2400|1200|600|300|110),popup(None|Even|Odd|Mark|Space),popup(5|6|7|8),popup(1|2),popup(64 deep|16 deep|1 deep),popup(1|quarter full|half full|almost full),checkbox,edit,popup(count+32 bit int|count+32 bit uint|count+16 bit int|count+16 bit uint|8 bit int null terminated|8 bit uint null terminated),edit,edit,edit,checkbox,edit,popup(count+32 bit int|count+32 bit uint|count+16 bit int|count+16 bit uint|8 bit int null terminated|8 bit uint null terminated),edit,popup(921600|460800|230400|115200|57600|38400|19200|9600|4800|2400|1200|600|300|110),popup(None|Even|Odd|Mark|Space),popup(5|6|7|8),popup(1|2),popup(64 deep|16 deep|1 deep),popup(1|quarter full|half full|almost full),checkbox,edit,popup(count+32 bit int|count+32 bit uint|count+16 bit int|count+16 bit uint|8 bit int null terminated|8 bit uint null terminated),edit,edit,edit,checkbox,edit,popup(count+32 bit int|count+32 bit uint|count+16 bit int|count+16 bit uint|8 bit int null terminated|8 bit uint null terminated),edit,popup(921600|460800|230400|115200|57600|38400|19200|9600|4800|2400|1200|600|300|110),popup(None|Even|Odd|Mark|Space),popup(5|6|7|8),popup(1|2),popup(64 deep|16 deep|1 deep),popup(1|quarter full|half full|almost full),checkbox,edit,popup(count+32 bit int|count+32 bit uint|count+16 bit int|count+16 bit uint|8 bit int null terminated|8 bit uint null terminated),edit,edit,edit,checkbox,edit,popup(count+32 bit int|count+32 bit uint|count+16 bit int|count+16 bit uint|8 bit int null terminated|8 bit uint null terminated),edit
      mask CallbackString:
      | mquamask( 2, 4 );
      | |mquamask( 2, 4 );||||||||||||||||||||||||||||||||||||||||||||||||||||||||||||||||||
      mask Display:
      | disp('QSC-100\n\nRS232\n\nSend Receive');
      | port_label( 'input', 1, 'XMT1' );
      | port_label( 'input', 2, 'XMT2' );
      | port_label( 'input', 3, 'XMT3' );
      | port_label( 'input', 4, 'XMT4' );
      | port_label( 'output', 1, 'RCV1' );
      | port_label( 'output', 2, 'RCV2' );
      | port_label( 'output', 3, 'RCV3' );
      | port_label( 'output', 4, 'RCV4' );
  QSC-100 Internal  blocks : Subsystem  PropExecContextAcrossSSBoundary=on
